simulink model "ex_3z1"  (R2018b)
settings: Solver=ode5  StartTime=0.0  StopTime=10  FixedStep=0.001  RelTol=1e-3
settings Model: Creator=ltiger  LastModifiedBy=QJ-
settings DebuggingCC: LibraryContextMissingDiagnostic=none
settings SFSimCC: SimUseLocalCustomCode=off
settings RTWCC: RTWUseLocalCustomCode=off
settings CodeAppCC: StateflowObjectComments=on

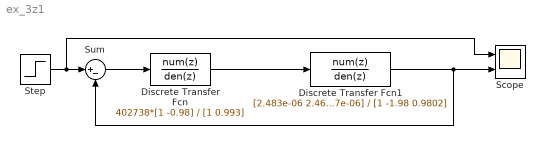
== system ex_3z1 ==
  Discrete Transfer Fcn : DiscreteTransferFcn  Numerator=402738*[1 -0.98]  Denominator=[1 0.993]  SampleTime=0.001
  Discrete Transfer Fcn1 : DiscreteTransferFcn  Numerator=[2.483e-06 2.467e-06]  Denominator=[1 -1.98 0.9802]  SampleTime=0.001
  Scope : Scope  NumInputPorts=2
  Step : Step  SampleTime=0.001  mask(DiscretizedSource){}
      mask init:
      | %zoh
  Sum : Sum  Inputs=|+-
  wires:
  Discrete Transfer Fcn/1 -> Discrete Transfer Fcn1/1
  Sum/1 -> Discrete Transfer Fcn/1
  Discrete Transfer Fcn1/1 -> Scope/2, Sum/2
  Step/1 -> Scope/1, Sum/1
